simulink model "xbox_controller_project_demo"  (R2025b)
settings: Solver=VariableStepAuto  StartTime=0.0  StopTime=10.0  RelTol=1e-3
model workspace (MAT data in the model file):
  mass = 0.543
  mmoi = 0.048
  moment_arm = 0.28
libraries: aerolibanim x1, aerolibanimutils x1
settings Model: Creator=Josh  LastModifiedBy=Josh

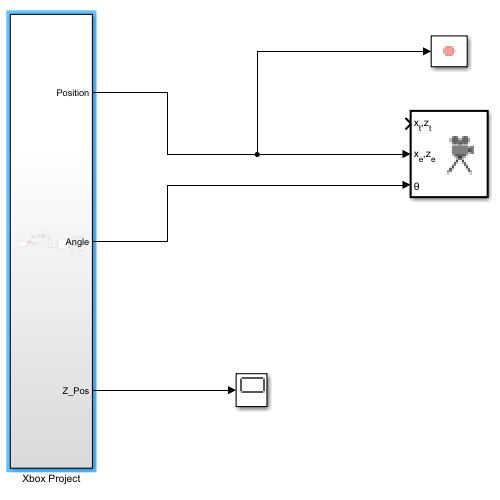
[thumbnail: Simulink's stored preview of the top-level diagram]
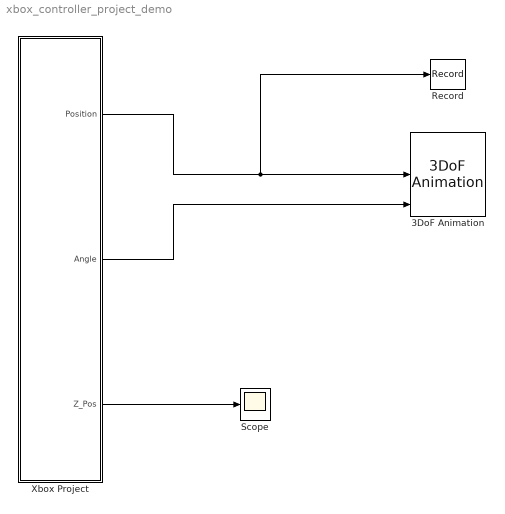
== system xbox_controller_project_demo ==
  3DoF Animation : aerolibanim/3DoF Animation  u1=[0 5000 -2000 2000 -5050 -3050]  u2=0.05  u3=1.0  u5=Fixed position  u6=[2000 500 -3150]  u7=10  u8=on
  Record : Record  NumPorts=1.0  FileSettingsInternal="{\"entries\":[{\"content\":{\"excelSettings\":{\"content\":{},\"type\":\"Streamout.ExcelSettings\"},\"parquetSettings\":{\"content\":{},\"type\":\"Streamout.ParquetSettings\"}},\"type\":\"Streamout.FileSettingStorage\",\"uuid\":\"\"}],\"packageUris\":[\"http:\\/\\/schema.mathworks.com\\/mf0\\/streamout_blocks\\/R2020a\"],\"version\":\"1.0\"}"  FrameSettings=0  Layout=[1 1]  SignalsInternal="{\"entries\":[{\"content\":{\"signals\":[{\"content\":{\"blockPath\":[],\"dimensions\":[2],\"domain\":\"\",\"hasChildren\":true,\"lineColor\":\"#ff6929\",\"lineWidth\":2,\"port\":1,\"signalID\":1,\"signalName\":\"Xbox Project:1\"},\"type\":\"RecordBlkView.Signal\",\"uuid\":\"\"},{\"content\":{\"blockPath\":[],\"channel\":[1],\"dimensions\":[2],\"domain\":\"\",\"lineColor\":\"#edb120\",\"lineWidth\":2,\"parentID\":1,\"plots\":[ 1 ],\"port\":1,\"signalID\":2,\"signalName\":\"Xbox Project:1\"},\"type\":\"RecordBlkView.Signal\",\"uuid\":\"\"},{\"content\":{\"blockPath\":[],\"channel\":[2],\"dimensions\":[2],\"domain\":\"\",\"lineColor\":\"#7e2f8e\",\"lineWidth\":2,\"parentID\":1,\"plots\":[ 1 ],\"port\":1,\"signalID\":3,\"signalName\":\"Xbox Project:1\"},\"type\":\"RecordBlkView.Signal\",\"uuid\":\"\"}]},\"type\":\"RecordBlkView.InputSignals\",\"uuid\":\"\"}],\"packageUris\":[\"http:\\/\\/schema.mathworks.com\\/mf0\\/streamout_blocks\\/R2020a\"],\"version\":\"1.0\"}"  VisualizationBindings="{\"xyplotplugin\":{\"info\":[{\"series\":[{\"bindingParametersList\":[{\"parameter\":\"X-Axis\",\"signalID\":2,\"signalName\":\"Xbox Project:1(1)\"},{\"parameter\":\"Y-Axis\",\"signalID\":3,\"signalName\":\"Xbox Project:1(2)\"}],\"seriesID\":0}],\"subplotID\":1}]}}"
  Scope : Scope
      settings: ActiveDisplayYMinimum=-353.33851832595383  ActiveDisplayYMaximum=1256.7776953054449
  Xbox Project : Subsystem
  wires:
  Xbox Project/1(Position) -> Record/1, 3DoF Animation/2
  Xbox Project/2(Angle) -> 3DoF Animation/3
  Xbox Project/3(Z_Pos) -> Scope/1

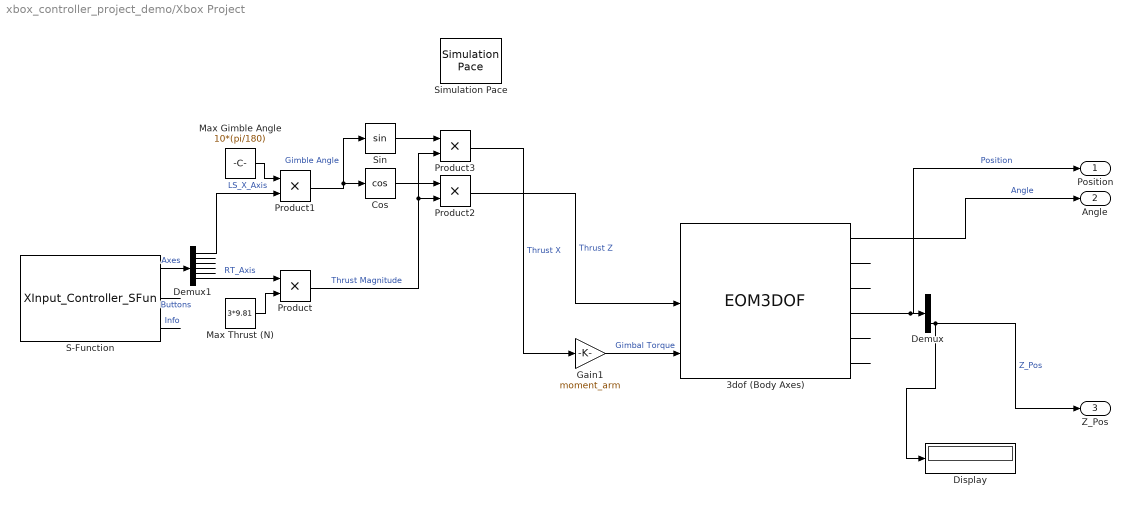
== system xbox_controller_project_demo/Xbox Project ==
  3dof (Body Axes) : EOM3DOF  v_ini=0  mass=mass  Iyy=mmoi  g=-9.81
  Cos : Trigonometry  Operator=cos
  Demux : Demux  Outputs=2
  Demux1 : Demux  Outputs=6
  Display : Display
  Gain1 : Gain  Gain=moment_arm
  Max Gimble Angle : Constant  Value=10*(pi/180)
  Max Thrust (N) : Constant  Value=3*9.81
  Product{,1..3} (4 alike) : Product
  S-Function : S-Function  FunctionName=XInput_Controller_SFun  Parameters=1  SFunctionDeploymentMode=off  EnableBusSupport=off
  Simulation Pace : aerolibanimutils/Simulation Pace  SimulationPace=1  SleepMode=Auto  OutputPaceError=off  SampleTime=1/30
  Sin : Trigonometry
  Position : Outport
  Angle : Outport  Port=2
  Z_Pos : Outport  Port=3
  wires:
  Demux1/1 -> Product1/2  "LS_X_Axis"
  Product2/1 -> 3dof (Body Axes)/2  "Thrust Z"
  Product3/1 -> Gain1/1  "Thrust X"
  3dof (Body Axes)/4 -> Position/1, Demux/1  "Position"
  Product1/1 -> Cos/1, Sin/1  "Gimble Angle"
  Max Thrust (N)/1 -> Product/2
  S-Function/1 -> Demux1/1  "Axes"
  Cos/1 -> Product2/1
  Max Gimble Angle/1 -> Product1/1
  Product/1 -> Product3/2, Product2/2  "Thrust Magnitude"
  Demux1/6 -> Product/1  "RT_Axis"
  Demux/2 -> Display/1, Z_Pos/1  "Z_Pos"
  Sin/1 -> Product3/1
  Gain1/1 -> 3dof (Body Axes)/3  "Gimbal Torque"
  3dof (Body Axes)/5 -> ?
  Demux1/2 -> ?
  3dof (Body Axes)/6 -> ?
  ? -> 3dof (Body Axes)/1
  3dof (Body Axes)/1 -> Angle/1  "Angle"
  Demux1/4 -> ?
  S-Function/3 -> ?  "Info"
  3dof (Body Axes)/2 -> ?
  Demux1/3 -> ?
  S-Function/2 -> ?  "Buttons"
  3dof (Body Axes)/3 -> ?
  Demux1/5 -> ?
